simulink model "zero_cross"  (R2021b)
settings: Solver=VariableStepAuto  StartTime=0.0  StopTime=10.0  RelTol=1e-3
undefined symbols (not defined in the file): Newton, Raphson
libraries: simulink x9
settings Model: PauseTimes=1  NumberOfSteps=5  Creator=cemery  LastModifiedBy=cemery
settings SolverCC: ZeroCrossAlgorithm=Adaptive  AlgebraicLoopSolver=TrustRegion
settings DataIOCC: ReturnWorkspaceOutputs=off
settings DebuggingCC: SFMachineParentedDataDiag=warning  ArithmeticOperatorsInVariantConditions=warning
settings SFSimCC: SimUseLocalCustomCode=off  CustomCodeUndefinedFunction=UseInterfaceOnly
settings RTWCC: RTWUseLocalCustomCode=off

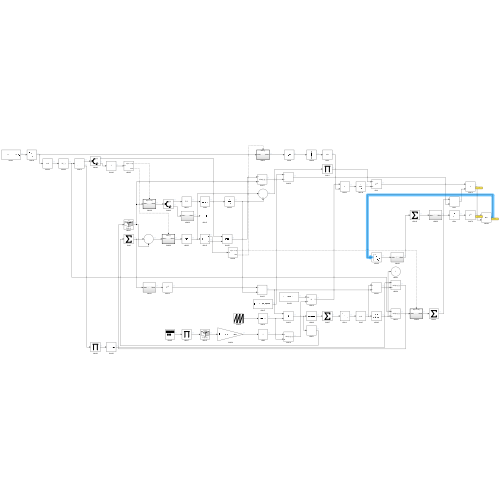
[thumbnail: Simulink's stored preview of the top-level diagram]
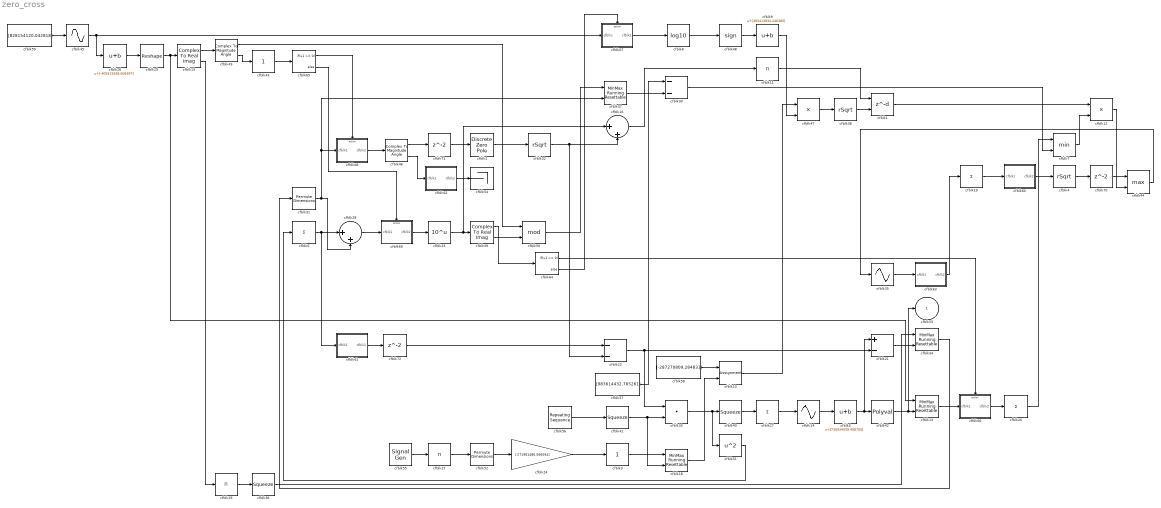
== system zero_cross ==
  cfblk1 : Delay  DelayLengthSource=Input port  SampleTime=1
      settings: InputPortMap=u0,p1
  cfblk10 : Assignment  DiagnosticForDimensions=Warning  IndexOptions=Index vector (dialog)  Indices=1  OutputSizes=1
  cfblk11 : Product  Inputs=*
  cfblk12 : Product  Inputs=**
  cfblk{13,18,34,37} (4 alike) : simulink/Math Operations/MinMax Running Resettable  Function=min  vinit=0.0
  cfblk14 : Sin  TimeSource=Use external signal  SampleTime=0
  cfblk15 : ComplexToRealImag
  cfblk16 : Sum  Inputs=|++
  cfblk17 : Product  Inputs=*
  cfblk{6,19..20,27} (4 alike) : Sum  Inputs=+
  cfblk2 : DiscreteZeroPole  Poles=[0 0.5]  Gain=1
  cfblk21 : Sum  Inputs=+-
  cfblk22 : Sum  Inputs=--
  cfblk23 : Math  Operator=10^u  SignedPower=on  SaturateOnIntegerOverflow=on
  cfblk24 : Gain  Gain=[-271961486.566094]
  cfblk25 : Reshape
  cfblk26 : Bias  Bias=[-405515938.608397]
  cfblk28 : Sum  Inputs=|++
  cfblk29 : Product  Inputs=*
  cfblk3 : simulink/Math Operations/Slider Gain  gain=1  low=0  high=2
  cfblk30 : Sum  Inputs=--
  cfblk31 : PermuteDimensions
  cfblk32 : Sqrt  Operator=rSqrt  AlgorithmType=Newton-Raphson  SaturateOnIntegerOverflow=on
  cfblk33 : DotProduct  InputSameDT=on  OutDataTypeStr=Inherit: Inherit via internal rule
  cfblk35 : Sin  TimeSource=Use external signal  SampleTime=0
  cfblk36 : Squeeze
  cfblk38 : Sqrt  Operator=rSqrt  AlgorithmType=Newton-Raphson  SaturateOnIntegerOverflow=on
  cfblk39 : ComplexToRealImag
  cfblk4 : Sqrt  Operator=rSqrt  AlgorithmType=Newton-Raphson  SaturateOnIntegerOverflow=on
  cfblk40 : Squeeze
  cfblk41 : Squeeze
  cfblk42 : Polyval  Coefs=[ +2.081618890e-019, -1.441693666e-014, +4.719686976e-010, -8.536869453e-006, +1.621573104e-001, -8.087801117e+001 ]
  cfblk43 : simulink/Math Operations/Slider Gain  gain=1  low=0  high=2
  cfblk44 : MinMax  Function=max  Inputs=2
  cfblk45 : Sin  TimeSource=Use external signal  SampleTime=0
  cfblk46 : ComplexToMagnitudeAngle
  cfblk47 : Product
  cfblk48 : Signum
  cfblk49 : ComplexToMagnitudeAngle
  cfblk5 : Bias  Bias=[730934059.458705]
  cfblk50 : Math  Operator=mod  SignedPower=on  SaturateOnIntegerOverflow=on
  cfblk51 : Math  Operator=square  SignedPower=on  SaturateOnIntegerOverflow=on
  cfblk52 : PermuteDimensions
  cfblk54 : Terminator
  cfblk55 : SignalGenerator  Amplitude=[-35271137.426169]
  cfblk56 : simulink/Sources/Repeating Sequence  rep_seq_t=[0 2]  rep_seq_y=[-297858002.361466, 698544900.369112]
  cfblk57 : Constant  Value=[983614432.765261]  SampleTime=1
  cfblk58 : Constant  Value=[-287270809.284831]  SampleTime=1
  cfblk59 : Constant  Value=[828154120.042818]  SampleTime=1
  cfblk60 : Subsystem
  cfblk61 : Subsystem
  cfblk62 : Subsystem
  cfblk63 : Subsystem
  cfblk64 : If  IfExpression=u1 >= 0  SampleTime=1
  cfblk65 : If  IfExpression=u1 >= 0  SampleTime=1
  cfblk66 : Subsystem  TreatAsAtomicUnit=on
  cfblk67 : Subsystem  TreatAsAtomicUnit=on
  cfblk68 : Subsystem  TreatAsAtomicUnit=on
  cfblk69 : Subsystem  TreatAsAtomicUnit=on
  cfblk7 : MinMax  Inputs=2
  cfblk70 : Delay  SampleTime=1
  cfblk71 : Delay  SampleTime=1
  cfblk72 : Delay  SampleTime=1
  cfblk8 : Math  Operator=log10  SignedPower=on  SaturateOnIntegerOverflow=on
  cfblk9 : Bias  Bias=[493413834.246385]
  cfblk53 : Outport  VectorParamsAs1DForOutWhenUnconnected=off
  wires:
  cfblk72/1 -> cfblk22/1
  cfblk15/2 -> cfblk29/1
  cfblk61/1(cfblk2) -> cfblk72/1
  cfblk4/1 -> cfblk70/1
  cfblk19/1 -> cfblk60/1(cfblk1)
  cfblk70/1 -> cfblk44/1
  cfblk11/1 -> cfblk1/1
  cfblk48/1 -> cfblk9/1
  cfblk46/1 -> cfblk71/1
  cfblk18/1 -> cfblk10/2
  cfblk71/1 -> cfblk2/1
  cfblk68/1(cfblk2) -> cfblk46/1
  cfblk65/1 -> cfblk68/Action
  cfblk13/1 -> cfblk66/1(cfblk1)
  cfblk52/1 -> cfblk24/1
  cfblk65/2 -> cfblk69/Action
  cfblk64/2 -> cfblk67/Action
  cfblk64/1 -> cfblk66/Action
  cfblk39/2 -> cfblk50/2
  cfblk58/1 -> cfblk10/1
  cfblk37/1 -> cfblk30/2
  cfblk30/1 -> cfblk7/2
  cfblk29/1 -> cfblk36/1
  cfblk50/1 -> cfblk37/1
  cfblk9/1 -> cfblk47/2
  cfblk21/1 -> cfblk34/2
  cfblk27/1 -> cfblk14/1
  cfblk39/1 -> cfblk64/1
  cfblk67/1(cfblk2) -> cfblk8/1
  cfblk46/2 -> cfblk62/1(cfblk1)
  cfblk49/1 -> cfblk50/1
  cfblk69/1(cfblk2) -> cfblk23/1
  cfblk66/1(cfblk2) -> cfblk20/1
  cfblk7/1 -> cfblk12/2
  cfblk44/1 -> cfblk35/1
  cfblk57/1 -> cfblk30/1
  cfblk51/1 -> cfblk6/1
  cfblk38/1 -> cfblk1/2
  cfblk36/1 -> cfblk34/1
  cfblk34/1 -> cfblk31/1
  cfblk43/1 -> cfblk65/1
  cfblk40/1 -> cfblk27/1
  cfblk28/1 -> cfblk69/1(cfblk1)
  cfblk16/1 -> cfblk11/1
  cfblk8/1 -> cfblk48/1
  cfblk10/1 -> cfblk47/1
  cfblk59/1 -> cfblk45/1
  cfblk12/1 -> cfblk44/2
  cfblk55/1 -> cfblk17/1
  cfblk49/2 -> cfblk43/1
  cfblk62/1(cfblk2) -> cfblk54/1
  cfblk2/1 -> cfblk32/1
  cfblk17/1 -> cfblk52/1
  cfblk26/1 -> cfblk25/1
  cfblk1/1 -> cfblk12/1
  cfblk24/1 -> cfblk3/1
  cfblk3/1 -> cfblk18/1
  cfblk60/1(cfblk2) -> cfblk4/1
  cfblk14/1 -> cfblk5/1
  cfblk35/1 -> cfblk63/1(cfblk1)
  cfblk15/1 -> cfblk49/1
  cfblk63/1(cfblk2) -> cfblk19/1
  cfblk47/1 -> cfblk38/1
  cfblk20/1 -> cfblk7/1
  cfblk56/1 -> cfblk41/1
  cfblk23/1 -> cfblk16/1, cfblk39/1
  cfblk45/1 -> cfblk26/1, cfblk67/1(cfblk1)
  cfblk42/1 -> cfblk53/1, cfblk13/2
  cfblk5/1 -> cfblk42/1, cfblk21/1
  cfblk22/1 -> cfblk33/1, cfblk21/2
  cfblk32/1 -> cfblk22/2, cfblk16/2
  cfblk25/1 -> cfblk15/1, cfblk13/1
  cfblk41/1 -> cfblk18/2, cfblk33/2
  cfblk33/1 -> cfblk40/1, cfblk51/1
  cfblk31/1 -> cfblk68/1(cfblk1), cfblk37/2, cfblk28/2
  cfblk6/1 -> cfblk61/1(cfblk1), cfblk28/1

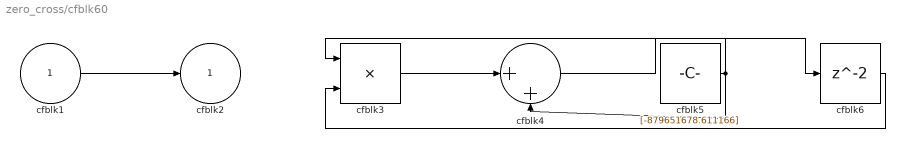
== system zero_cross/cfblk60 ==
  cfblk1 : Inport
  cfblk3 : Product
  cfblk4 : Sum  Inputs=|++
  cfblk5 : Constant  Value=[-879651678.611166]  SampleTime=1
  cfblk6 : Delay  SampleTime=1
  cfblk2 : Outport  VectorParamsAs1DForOutWhenUnconnected=off
  wires:
  cfblk1/1 -> cfblk2/1
  cfblk5/1 -> cfblk3/1, cfblk4/2
  cfblk3/1 -> cfblk4/1
  cfblk4/1 -> cfblk6/1
  cfblk6/1 -> cfblk3/2

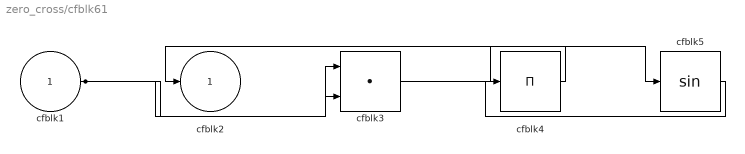
== system zero_cross/cfblk61 ==
  cfblk1 : Inport
  cfblk3 : DotProduct  InputSameDT=on  OutDataTypeStr=Inherit: Inherit via internal rule
  cfblk4 : Product  Inputs=*
  cfblk5 : Trigonometry
  cfblk2 : Outport  VectorParamsAs1DForOutWhenUnconnected=off
  wires:
  cfblk3/1 -> cfblk5/1
  cfblk5/1 -> cfblk4/1
  cfblk4/1 -> cfblk2/1
  cfblk1/1 -> cfblk3/1, cfblk3/2

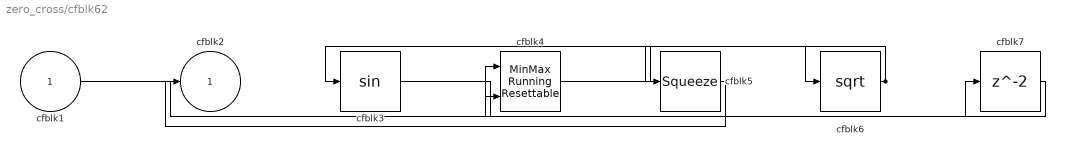
== system zero_cross/cfblk62 ==
  cfblk1 : Inport
  cfblk3 : Trigonometry
  cfblk4 : simulink/Math Operations/MinMax Running Resettable  Function=min  vinit=0.0
  cfblk5 : Squeeze
  cfblk6 : Sqrt  SaturateOnIntegerOverflow=on
  cfblk7 : Delay  SampleTime=1
  cfblk2 : Outport  VectorParamsAs1DForOutWhenUnconnected=off
  wires:
  cfblk6/1 -> cfblk3/1, cfblk5/1
  cfblk1/1 -> cfblk4/1
  cfblk5/1 -> cfblk2/1
  cfblk4/1 -> cfblk6/1
  cfblk3/1 -> cfblk7/1
  cfblk7/1 -> cfblk4/2

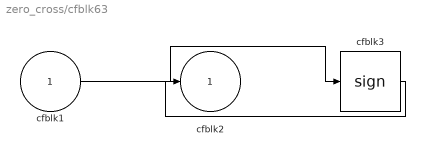
== system zero_cross/cfblk63 ==
  cfblk1 : Inport
  cfblk3 : Signum
  cfblk2 : Outport  VectorParamsAs1DForOutWhenUnconnected=off
  wires:
  cfblk1/1 -> cfblk3/1
  cfblk3/1 -> cfblk2/1

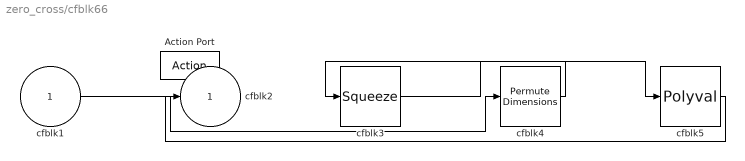
== system zero_cross/cfblk66 ==
  cfblk1 : Inport
  Action Port : ActionPort  ActionPortLabel=if(u1 >= 0)
  cfblk3 : Squeeze
  cfblk4 : PermuteDimensions
  cfblk5 : Polyval  Coefs=[ +2.081618890e-019, -1.441693666e-014, +4.719686976e-010, -8.536869453e-006, +1.621573104e-001, -8.087801117e+001 ]
  cfblk2 : Outport  VectorParamsAs1DForOutWhenUnconnected=off
  wires:
  cfblk4/1 -> cfblk3/1
  cfblk1/1 -> cfblk4/1
  cfblk3/1 -> cfblk5/1
  cfblk5/1 -> cfblk2/1

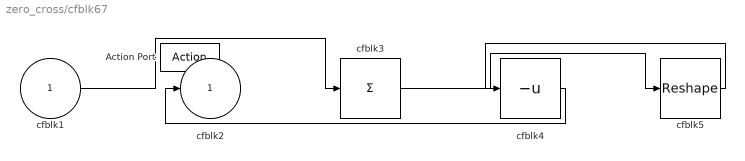
== system zero_cross/cfblk67 ==
  cfblk1 : Inport
  Action Port : ActionPort  ActionPortLabel=else
  cfblk3 : Sum  Inputs=+
  cfblk4 : UnaryMinus
  cfblk5 : Reshape
  cfblk2 : Outport  VectorParamsAs1DForOutWhenUnconnected=off
  wires:
  cfblk4/1 -> cfblk2/1
  cfblk1/1 -> cfblk3/1
  cfblk3/1 -> cfblk5/1
  cfblk5/1 -> cfblk4/1

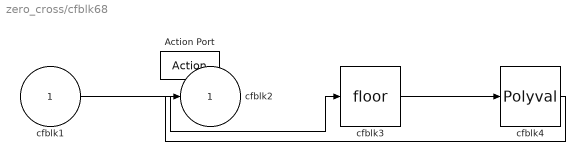
== system zero_cross/cfblk68 ==
  cfblk1 : Inport
  Action Port : ActionPort  ActionPortLabel=if(u1 >= 0)
  cfblk3 : Rounding
  cfblk4 : Polyval  Coefs=[ +2.081618890e-019, -1.441693666e-014, +4.719686976e-010, -8.536869453e-006, +1.621573104e-001, -8.087801117e+001 ]
  cfblk2 : Outport  VectorParamsAs1DForOutWhenUnconnected=off
  wires:
  cfblk1/1 -> cfblk3/1
  cfblk4/1 -> cfblk2/1
  cfblk3/1 -> cfblk4/1

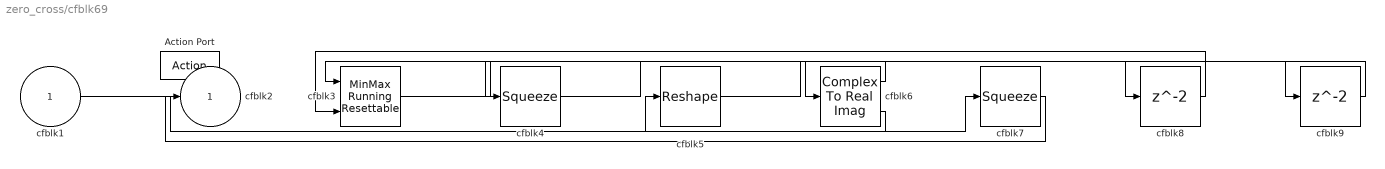
== system zero_cross/cfblk69 ==
  cfblk1 : Inport
  Action Port : ActionPort  ActionPortLabel=else
  cfblk3 : simulink/Math Operations/MinMax Running Resettable  Function=min  vinit=0.0
  cfblk4 : Squeeze
  cfblk5 : Reshape
  cfblk6 : ComplexToRealImag
  cfblk7 : Squeeze
  cfblk8 : Delay
  cfblk9 : Delay
  cfblk2 : Outport  VectorParamsAs1DForOutWhenUnconnected=off
  wires:
  cfblk1/1 -> cfblk7/1
  cfblk3/1 -> cfblk6/1
  cfblk7/1 -> cfblk2/1
  cfblk6/1 -> cfblk4/1
  cfblk6/2 -> cfblk5/1
  cfblk4/1 -> cfblk8/1
  cfblk8/1 -> cfblk3/2
  cfblk5/1 -> cfblk9/1
  cfblk9/1 -> cfblk3/1
